simulink model "BMS_software"  (R2023b)
settings: Solver=VariableStepAuto  StartTime=0.0  StopTime=Inf  RelTol=1e-3  EnableMultiTasking=on
settings Model: DataDictionary=OurShared_DD.sldd  EnableAccessToBaseWorkspace=off  ExtModeTrigDuration=8  Creator=Alkhouly  LastModifiedBy=Alkhouly

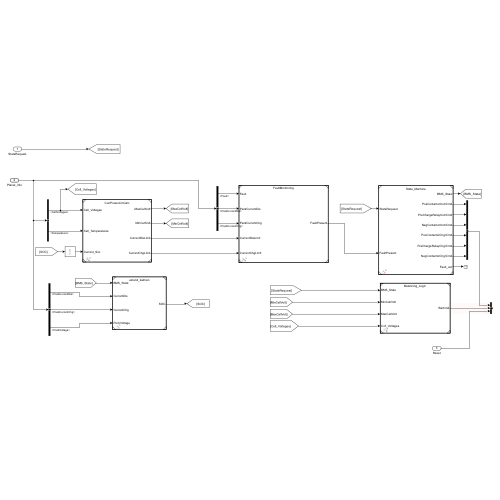
[thumbnail: Simulink's stored preview of the top-level diagram]
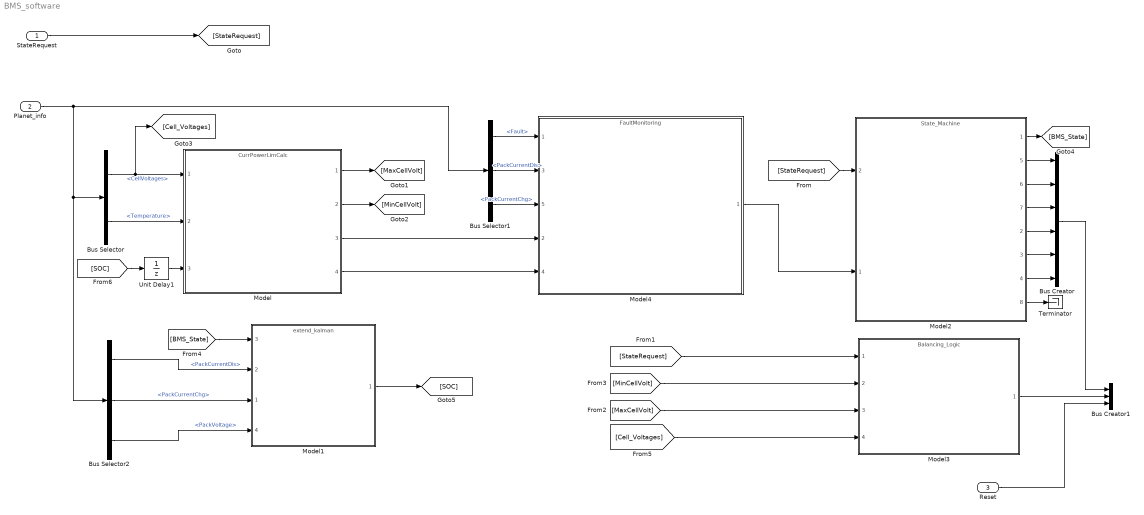
== system BMS_software ==
  StateRequest : Inport
  Planet_info : Inport  Port=2  OutDataTypeStr=Bus: BMS_input
  Reset : Inport  Port=3
  Bus Creator : BusCreator  Inputs=6  OutDataTypeStr=Bus: SwitcingCommands
  Bus Creator1 : BusCreator  Inputs=3  OutDataTypeStr=Bus: From_BMS
  Bus Selector : BusSelector  OutputSignals=CellVoltages,Temperature
  Bus Selector1 : BusSelector  OutputSignals=Fault,PackCurrentDis,PackCurrentChg
  Bus Selector2 : BusSelector  OutputSignals=PackCurrentDis,PackCurrentChg,PackVoltage
  Model : ModelReference  ModelNameDialog=CurrPowerLimCalc.slx  SimulationMode=Normal  ModelReferenceVersion=10.1
  Model1 : ModelReference  ModelNameDialog=extend_kalman.slx  SimulationMode=Normal  ModelReferenceVersion=6.8
      settings: PortSchema="{\"entries\":[{\"content\":{\"sides\":[{\"content\":{\"connectorIds\":[\"In3\",\"In2\",\"In1\",\"In4\"]},\"type\":\"ConnectorPlacement.EquallySpacedRectSide\",\"uuid\":\"df0417c6-f4f4-4b55-abd2-d25cd88120da\"},{\"content\":{\"connectorIds\":[\"Out1\"],\"side\":\"RIGHT\"},\"type\":\"ConnectorPlacement.EquallySpacedRectSide\",\"uuid\":\"aa17d75f-49b6-4d16-ad89-5d6fe3e04eb1\"},{\"content\":{\"side\":\"TOP\"},\"type\":\"ConnectorPlacement.EquallySpacedRectSide\",\"uuid\":\"fae0d4ff-403f-4ff6-b763-7c4f268d8f7f\"}]},\"type\":\"ConnectorPlacement.EquallySpacedConnector\",\"uuid\":\"adc2ca63-742b-4f39-aef4-0160e2e61c03\"}],\"packageUris\":[\"http://schema.mathworks.com/mf0/Connector/R2020b\"],\"version\":\"1.0\"}"
  Model2 : ModelReference  ModelNameDialog=State_Machine.slx  SimulationMode=Normal  ModelReferenceVersion=9.16
      settings: PortSchema="{\"entries\":[{\"content\":{\"sides\":[{\"content\":{\"connectorIds\":[\"In2\",\"In1\"]},\"type\":\"ConnectorPlacement.EquallySpacedRectSide\",\"uuid\":\"a6321078-a11a-4ff4-ac46-fc5269a50794\"},{\"content\":{\"connectorIds\":[\"Out1\",\"Out5\",\"Out6\",\"Out7\",\"Out2\",\"Out3\",\"Out4\",\"Out8\"],\"side\":\"RIGHT\"},\"type\":\"ConnectorPlacement.EquallySpacedRectSide\",\"uuid\":\"cec00c8d-93c5-45b2-be42-b1bc8b9d3d24\"},{\"content\":{\"side\":\"TOP\"},\"type\":\"ConnectorPlacement.EquallySpacedRectSide\",\"uuid\":\"565557e9-1b71-4c6f-9d05-1c346465bf3f\"}]},\"type\":\"ConnectorPlacement.EquallySpacedConnector\",\"uuid\":\"c691f22a-3ebe-4ca0-a8f4-8866b2ce5f7f\"}],\"packageUris\":[\"http://schema.mathworks.com/mf0/Connector/R2020b\"],\"version\":\"1.0\"}"
  Model3 : ModelReference  ModelNameDialog=Balancing_Logic.slx  SimulationMode=Normal  ModelReferenceVersion=9.4
  Model4 : ModelReference  ModelNameDialog=FaultMonitoring.slx  SimulationMode=Normal  ModelReferenceVersion=1.3
      settings: PortSchema="{\"entries\":[{\"content\":{\"sides\":[{\"content\":{\"connectorIds\":[\"In1\",\"In3\",\"In5\",\"In2\",\"In4\"]},\"type\":\"ConnectorPlacement.EquallySpacedRectSide\",\"uuid\":\"0f409363-c677-4444-b3b4-70125efc82aa\"},{\"content\":{\"connectorIds\":[\"Out1\"],\"side\":\"RIGHT\"},\"type\":\"ConnectorPlacement.EquallySpacedRectSide\",\"uuid\":\"cf9a1433-f278-49df-a32e-2d15abcd8f19\"},{\"content\":{\"side\":\"TOP\"},\"type\":\"ConnectorPlacement.EquallySpacedRectSide\",\"uuid\":\"6fb8c4a4-1a26-4c65-88a8-7de305e54a21\"}]},\"type\":\"ConnectorPlacement.EquallySpacedConnector\",\"uuid\":\"cdc8a9ef-2c4b-46f2-b943-79d24cd71111\"}],\"packageUris\":[\"http://schema.mathworks.com/mf0/Connector/R2020b\"],\"version\":\"1.0\"}"
  Terminator : Terminator
  Unit Delay1 : UnitDelay  SampleTime=-1  HasFrameUpgradeWarning=on
  wires:
  Planet_info/1 -> Bus Selector/1, Bus Selector2/1, Bus Selector1/1
  Bus Selector/1 -> [Cell_Voltages], Model/1  "<CellVoltages>"
  Bus Selector/2 -> Model/2  "<Temperature>"
  Model/3 -> Model4/2
  Model/4 -> Model4/4
  Bus Selector1/1 -> Model4/1  "<Fault>"
  Bus Selector1/2 -> Model4/3  "<PackCurrentDis>"
  Bus Selector1/3 -> Model4/5  "<PackCurrentChg>"
  Model4/1 -> Model2/1
  StateRequest/1 -> [StateRequest]
  [StateRequest] -> Model2/2
  [StateRequest] -> Model3/1
  Model/1 -> [MaxCellVolt]
  Model/2 -> [MinCellVolt]
  [MaxCellVolt] -> Model3/3
  [MinCellVolt] -> Model3/2
  [Cell_Voltages] -> Model3/4
  Bus Selector2/3 -> Model1/4  "<PackVoltage>"
  Bus Selector2/1 -> Model1/2  "<PackCurrentDis>"
  Bus Selector2/2 -> Model1/1  "<PackCurrentChg>"
  Model2/8 -> Terminator/1
  [BMS_State] -> Model1/3
  Model1/1 -> [SOC]
  Unit Delay1/1 -> Model/3
  [SOC] -> Unit Delay1/1
  Model2/5 -> Bus Creator/1
  Model2/6 -> Bus Creator/2
  Model2/7 -> Bus Creator/3
  Model2/2 -> Bus Creator/4
  Model2/3 -> Bus Creator/5
  Model2/4 -> Bus Creator/6
  Bus Creator/1 -> Bus Creator1/1
  Model2/1 -> [BMS_State]
  Model3/1 -> Bus Creator1/2
  Reset/1 -> Bus Creator1/3
